simulink model "p2semanti"  (R2020a)
settings: Solver=VariableStepAuto  StartTime=0.0  StopTime=5  RelTol=1e-3
values from neighbouring files (symbols this model uses):
  B = 0.003032    [motorfase_valores.m]
  flux = 0.12    [motorfase_valores.m]
  inddiff = 0.0125    [motorfase_valores.m]
  J = 0.0042    [motorfase_valores.m]
  p = 3    [motorfase_valores.m]
  R = 2.3    [motorfase_valores.m]
undefined symbols (not defined in the file or in its folder): Down, Up
libraries: powerlib x13, eePwmGenerator x1, simulink x1
settings Model: Creator=ryt14  LastModifiedBy=ryt14

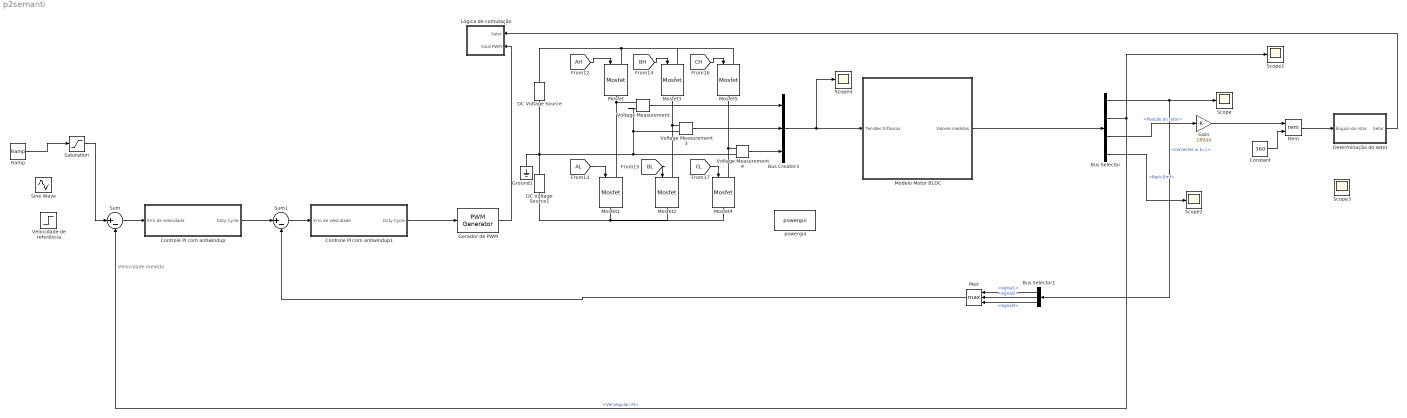
== system p2semanti ==
  note: Velocidade medida
  Bus Creator3 : BusCreator  Inputs=3
  Bus Selector : BusSelector  OutputSignals=Correntes a; b; c,Vel angular: PI,Posição do rotor,Back-Emf
  Bus Selector1 : BusSelector  OutputSignals=signal1,signal2,signal3
  Constant : Constant  Value=360
  Controle PI com antiwindup : Subsystem
  Controle PI com antiwindup1 : Subsystem
  DC Voltage Source : powerlib/Electrical Sources/DC Voltage Source  Amplitude=75  Measurements=None
  DC Voltage Source1 : powerlib/Electrical Sources/DC Voltage Source  Amplitude=75  Measurements=None
  Determinação do setor : Subsystem
  Gain : Gain  Gain=180/pi
  Gerador de PWM : eePwmGenerator/PWM Generator  CarrCount=Up-Down  Tper=0.001  Ts=5e-5
  Ground1 : powerlib/Elements/Ground  LConnTagsString=a
  Lógica de comutação : Subsystem
  Max : MinMax  Function=max  Inputs=3
  Modelo Motor BLDC : Subsystem
  Mosfet{,1..5} (6 alike) : powerlib/Power Electronics/Mosfet  Ron=0.1  Lon=0  Rd=0.01  Vfd=0  IC=0  Rs=1e5  Cs=inf  Measurements=off
  Ramp : simulink/Sources/Ramp  slope=50  start=0  InitialOutput=0
  Rem : Math  Operator=rem  SaturateOnIntegerOverflow=on
  Saturation : Saturate  UpperLimit=100  LowerLimit=0
  Scope{,1..4} (5 alike) : Scope
  Sine Wave : Sin  Amplitude=100  Frequency=pi/5  SampleTime=0
  Sum : Sum  Inputs=|+-
  Sum1 : Sum  Inputs=|+-
  Velocidade de referência : Step  Time=0  After=50  SampleTime=0
  Voltage Measurement : powerlib/Measurements/Voltage Measurement  PhasorSimulation=off  OutputType=Complex  PSBequivalent=0
  Voltage Measurement3 : powerlib/Measurements/Voltage Measurement  PhasorSimulation=off  OutputType=Complex  PSBequivalent=0
  Voltage Measurement4 : powerlib/Measurements/Voltage Measurement  PhasorSimulation=off  OutputType=Complex  PSBequivalent=0
  powergui : powerlib/powergui  Priority=1  SimulationMode=Continuous  SampleTime=50e-6  frequency=60  Iterations=50  frequencyindice=0  Pbase=100e6  ErrMax=1e-4  UnitsV=kV  UnitsW=MW  buscounter=0  FunctionMessages=off  echomessages=off  EnableUseOfTLC=off  CurrentSourceSwitches=off  DisableSnubberDevices=off  DisableRonSwitches=off  DisableVfSwitches=off  DisplayEquations=off  AutomaticDiscreteSolvers=off  SolverType=Tustin/Backward Euler (TBE)  Interpol=off  ExternalGateDelay=off  methode=off  Ts=100  x0status=blocks  SPID=on  SwTol=0  HookPort=off  NonlinearTolerance=1e-4  nMaxIteration=100  ContinueOnMaxIteration=off  RestoreLinks=warning  ResistiveCurrentMeasurement=off  Frange=[0:2:500]  Ylog=off  Xlog=on  ShowGrid=off  save=off  variable=ZData  structure=0  ZoomFFT=off  StartTime=0.0  cycles=1  DisplayStyle=1  fundamental=60  FreqAxis=off  MaxFrequency=1000  frequencyindicesteady=1  RmsSteady=1  display=off
  wires:
  Voltage Measurement3/1 -> Bus Creator3/2
  Voltage Measurement4/1 -> Bus Creator3/3
  Voltage Measurement/1 -> Bus Creator3/1
  Modelo Motor BLDC/1(Valores medidos) -> Bus Selector/1
  Gain/1 -> Rem/1
  Bus Selector/3 -> Gain/1  "<Posição do rotor>"
  Constant/1 -> Rem/2
  Rem/1 -> Determinação do setor/1(Ângulo do rotor)
  Bus Selector/2 -> Sum/2, Scope1/1  "<Vel angular: PI>"
  [AH] -> Mosfet/1
  [BH] -> Mosfet3/1
  [CH] -> Mosfet5/1
  [BL] -> Mosfet2/1
  [CL] -> Mosfet4/1
  [AL] -> Mosfet1/1
  Bus Selector/1 -> Bus Selector1/1, Scope/1  "<Correntes a; b; c>"
  Bus Selector/4 -> Scope2/1  "<Back-Emf>"
  Determinação do setor/1(Setor) -> Lógica de comutação/1(Setor)
  Gerador de PWM/1 -> Lógica de comutação/2(Sinal PWM)
  Sum/1 -> Controle PI com antiwindup/1(Erro de velocidade)
  Bus Creator3/1 -> Scope4/1, Modelo Motor BLDC/1(Tensões trifásicas)
  Bus Selector1/1 -> Max/1  "<signal1>"
  Bus Selector1/2 -> Max/2  "<signal2>"
  Bus Selector1/3 -> Max/3  "<signal3>"
  Sum1/1 -> Controle PI com antiwindup1/1(Erro de velocidade)
  Max/1 -> Sum1/2
  Controle PI com antiwindup/1(Duty Cycle) -> Sum1/1
  Controle PI com antiwindup1/1(Duty Cycle) -> Gerador de PWM/1
  Ramp/1 -> Saturation/1
  Saturation/1 -> Sum/1
  connections:
  Mosfet/RConn1 -- Mosfet1/LConn1 -- Voltage Measurement/LConn1
  Mosfet3/RConn1 -- Mosfet2/LConn1 -- Voltage Measurement3/LConn1
  Mosfet5/RConn1 -- Mosfet4/LConn1 -- Voltage Measurement4/LConn1
  Mosfet/LConn1 -- Mosfet5/LConn1 -- Mosfet3/LConn1 -- DC Voltage Source/RConn1
  DC Voltage Source/LConn1 -- Voltage Measurement4/LConn2 -- Voltage Measurement3/LConn2 -- Voltage Measurement/LConn2 -- Ground1/LConn1 -- DC Voltage Source1/RConn1
  Mosfet4/RConn1 -- Mosfet2/RConn1 -- DC Voltage Source1/LConn1 -- Mosfet1/RConn1

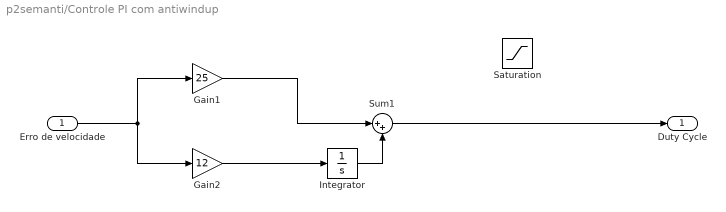
== system p2semanti/Controle PI com antiwindup ==
  Erro de velocidade : Inport
  Gain1 : Gain  Gain=25
  Gain2 : Gain  Gain=12
  Integrator : Integrator
  Saturation : Saturate
  Sum1 : Sum  Inputs=|++
  Duty Cycle : Outport
  wires:
  Integrator/1 -> Sum1/2
  Gain1/1 -> Sum1/1
  Erro de velocidade/1 -> Gain1/1, Gain2/1
  Sum1/1 -> Duty Cycle/1
  Gain2/1 -> Integrator/1

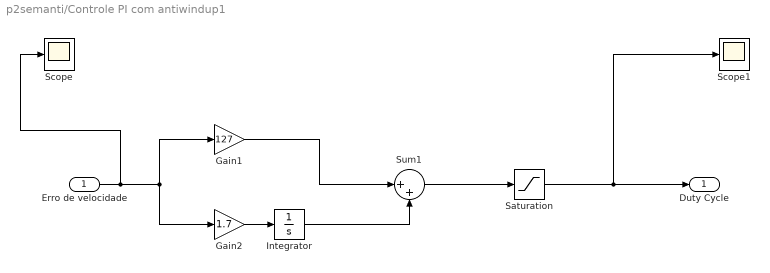
== system p2semanti/Controle PI com antiwindup1 ==
  Erro de velocidade : Inport
  Gain1 : Gain  Gain=127
  Gain2 : Gain  Gain=1.7
  Integrator : Integrator
  Saturation : Saturate  UpperLimit=1  LowerLimit=0
  Scope : Scope
  Scope1 : Scope
  Sum1 : Sum  Inputs=|++
  Duty Cycle : Outport
  wires:
  Sum1/1 -> Saturation/1
  Erro de velocidade/1 -> Scope/1, Gain1/1, Gain2/1
  Saturation/1 -> Scope1/1, Duty Cycle/1
  Gain2/1 -> Integrator/1
  Integrator/1 -> Sum1/2
  Gain1/1 -> Sum1/1

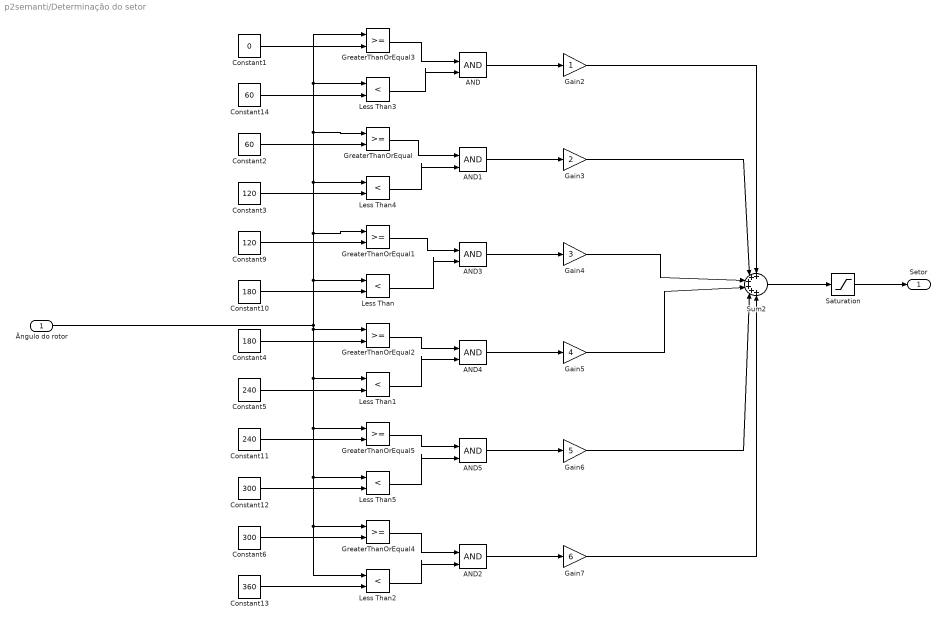
== system p2semanti/Determinação do setor ==
  Ângulo do rotor : Inport
  AND{,1..5} (6 alike) : Logic  IconShape=distinctive  AllPortsSameDT=off  OutDataTypeStr=boolean
  Constant1 : Constant  Value=0
  Constant10 : Constant  Value=180
  Constant11 : Constant  Value=240
  Constant12 : Constant  Value=300
  Constant13 : Constant  Value=360
  Constant14 : Constant  Value=60
  Constant2 : Constant  Value=60
  Constant3 : Constant  Value=120
  Constant4 : Constant  Value=180
  Constant5 : Constant  Value=240
  Constant6 : Constant  Value=300
  Constant9 : Constant  Value=120
  Gain2 : Gain
  Gain3 : Gain  Gain=2
  Gain4 : Gain  Gain=3
  Gain5 : Gain  Gain=4
  Gain6 : Gain  Gain=5
  Gain7 : Gain  Gain=6
  GreaterThanOrEqual{,1..5} (6 alike) : RelationalOperator  OutDataTypeStr=boolean  RndMeth=Simplest
  Less Than{,1..5} (6 alike) : RelationalOperator  Operator=<  OutDataTypeStr=boolean  RndMeth=Simplest
  Saturation : Saturate  UpperLimit=6  LowerLimit=1
  Sum2 : Sum  Inputs=++++++
  Setor : Outport
  wires:
  Ângulo do rotor/1 -> Less Than/1, GreaterThanOrEqual1/1, GreaterThanOrEqual/1, GreaterThanOrEqual3/1, Less Than3/1, Less Than4/1, Less Than2/1, GreaterThanOrEqual4/1, Less Than5/1, GreaterThanOrEqual5/1, Less Than1/1, GreaterThanOrEqual2/1
  Less Than1/1 -> AND4/2
  Gain2/1 -> Sum2/1
  Sum2/1 -> Saturation/1
  Constant1/1 -> GreaterThanOrEqual3/2
  Constant9/1 -> GreaterThanOrEqual1/2
  Gain4/1 -> Sum2/3
  Gain5/1 -> Sum2/4
  AND/1 -> Gain2/1
  Constant13/1 -> Less Than2/2
  Constant2/1 -> GreaterThanOrEqual/2
  AND4/1 -> Gain5/1
  AND1/1 -> Gain3/1
  Less Than5/1 -> AND5/2
  Less Than/1 -> AND3/2
  GreaterThanOrEqual1/1 -> AND3/1
  Constant4/1 -> GreaterThanOrEqual2/2
  Gain3/1 -> Sum2/2
  Less Than2/1 -> AND2/2
  GreaterThanOrEqual5/1 -> AND5/1
  GreaterThanOrEqual/1 -> AND1/1
  Gain6/1 -> Sum2/5
  AND2/1 -> Gain7/1
  AND5/1 -> Gain6/1
  Less Than3/1 -> AND/2
  Constant11/1 -> GreaterThanOrEqual5/2
  Constant12/1 -> Less Than5/2
  Constant3/1 -> Less Than4/2
  Constant5/1 -> Less Than1/2
  Saturation/1 -> Setor/1
  AND3/1 -> Gain4/1
  Constant14/1 -> Less Than3/2
  GreaterThanOrEqual2/1 -> AND4/1
  Less Than4/1 -> AND1/2
  Constant6/1 -> GreaterThanOrEqual4/2
  Constant10/1 -> Less Than/2
  GreaterThanOrEqual4/1 -> AND2/1
  Gain7/1 -> Sum2/6
  GreaterThanOrEqual3/1 -> AND/1

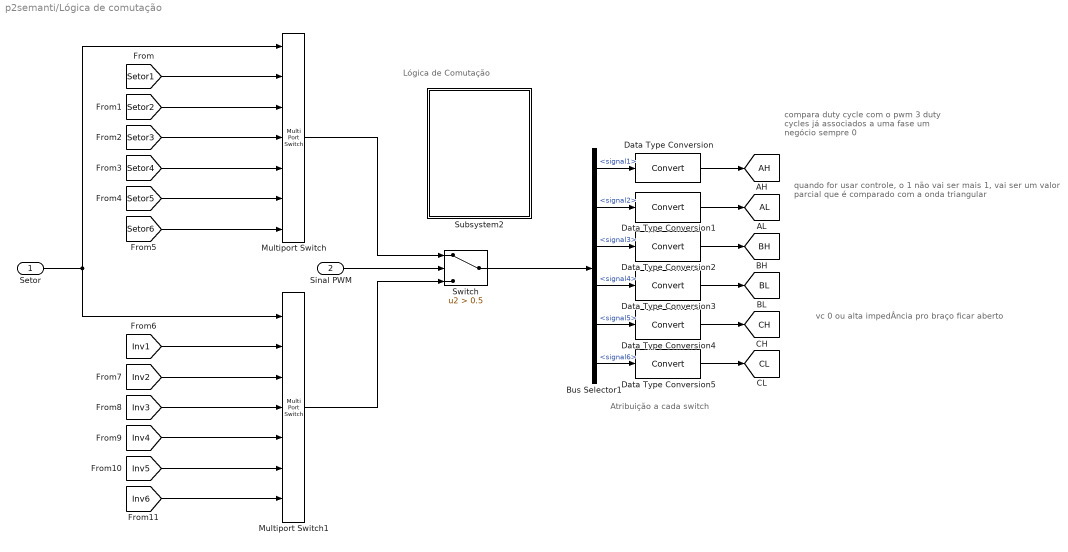
== system p2semanti/Lógica de comutação ==
  note: vc 0 ou alta impedÂncia pro braço ficar aberto
  note: quando for usar controle, o 1 não vai ser mais 1,
      | vai ser um valor parcial que é comparado com a onda triangular
  note: compara duty cycle com o pwm
      | 3 duty cycles já associados a uma fase
      | um negócio sempre 0
  note: Atribuição a cada switch
  note: Lógica de Comutação
  Setor : Inport
  Sinal PWM : Inport  Port=2
  Bus Selector1 : BusSelector  OutputSignals=signal1,signal2,signal3,signal4,signal5,signal6
  Data Type Conversion{,1..5} (6 alike) : DataTypeConversion
  Multiport Switch : MultiPortSwitch  Inputs=6
  Multiport Switch1 : MultiPortSwitch  Inputs=6
  Subsystem2 : Subsystem
  Switch : Switch  Criteria=u2 > Threshold  Threshold=0.5
  tag scope: AH=global, AL=global, BH=global, BL=global, CH=global, CL=global
  wires:
  [Inv4] -> Multiport Switch1/5
  Data Type Conversion5/1 -> [CL]
  [Setor1] -> Multiport Switch/2
  Bus Selector1/2 -> Data Type Conversion1/1  "<signal2>"
  Bus Selector1/4 -> Data Type Conversion3/1  "<signal4>"
  Data Type Conversion4/1 -> [CH]
  [Setor2] -> Multiport Switch/3
  [Inv1] -> Multiport Switch1/2
  Data Type Conversion1/1 -> [AL]
  Bus Selector1/3 -> Data Type Conversion2/1  "<signal3>"
  [Setor3] -> Multiport Switch/4
  [Inv3] -> Multiport Switch1/4
  Data Type Conversion3/1 -> [BL]
  [Setor5] -> Multiport Switch/6
  Switch/1 -> Bus Selector1/1
  Multiport Switch/1 -> Switch/1
  Bus Selector1/1 -> Data Type Conversion/1  "<signal1>"
  [Inv5] -> Multiport Switch1/6
  [Inv6] -> Multiport Switch1/7
  Bus Selector1/6 -> Data Type Conversion5/1  "<signal6>"
  [Inv2] -> Multiport Switch1/3
  Setor/1 -> Multiport Switch/1, Multiport Switch1/1
  Data Type Conversion/1 -> [AH]
  Bus Selector1/5 -> Data Type Conversion4/1  "<signal5>"
  [Setor4] -> Multiport Switch/5
  Data Type Conversion2/1 -> [BH]
  Multiport Switch1/1 -> Switch/3
  [Setor6] -> Multiport Switch/7
  Sinal PWM/1 -> Switch/2

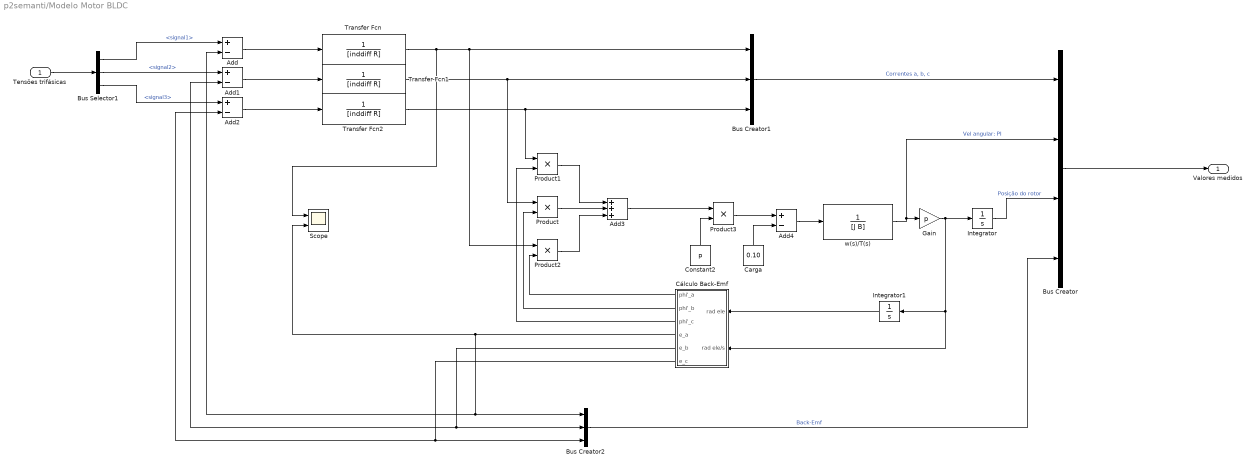
== system p2semanti/Modelo Motor BLDC ==
  Tensões trifásicas : Inport
  Add{,1..2,4} (4 alike) : Sum  Inputs=+-
  Add3 : Sum  Inputs=+++
  Bus Creator : BusCreator  Inputs=4
  Bus Creator1 : BusCreator  Inputs=3
  Bus Creator2 : BusCreator  Inputs=3
  Bus Selector1 : BusSelector  OutputSignals=signal1,signal2,signal3
  Carga : Constant  Value=0.10
  Constant2 : Constant  Value=p
  Cálculo Back-Emf : Subsystem
  Gain : Gain  Gain=p
  Integrator : Integrator
  Integrator1 : Integrator
  Product : Product
  Product1 : Product
  Product2 : Product
  Product3 : Product  Inputs=**
  Scope : Scope  NumInputPorts=2
  Transfer Fcn : TransferFcn  Denominator=[inddiff R]
  Transfer Fcn1 : TransferFcn  Denominator=[inddiff R]
  Transfer Fcn2 : TransferFcn  Denominator=[inddiff R]
  w(s)/T(s) : TransferFcn  Denominator=[J B]
  Valores medidos : Outport
  wires:
  Add/1 -> Transfer Fcn/1
  Add2/1 -> Transfer Fcn2/1
  Carga/1 -> Add4/2
  Bus Selector1/2 -> Add1/1  "<signal2>"
  Bus Creator1/1 -> Bus Creator/1  "Correntes a, b, c"
  Add1/1 -> Transfer Fcn1/1
  Transfer Fcn1/1 -> Bus Creator1/2, Product/1
  Product3/1 -> Add4/1
  Bus Selector1/1 -> Add/1  "<signal1>"
  Transfer Fcn2/1 -> Bus Creator1/3, Product1/1
  Add4/1 -> w(s)/T(s)/1
  Transfer Fcn/1 -> Scope/1, Bus Creator1/1, Product2/1
  Bus Selector1/3 -> Add2/1  "<signal3>"
  Bus Creator2/1 -> Bus Creator/4  "Back-Emf"
  Product/1 -> Add3/2
  Tensões trifásicas/1 -> Bus Selector1/1
  Gain/1 -> Integrator/1, Cálculo Back-Emf/2(rad ele/s), Integrator1/1
  Integrator/1 -> Bus Creator/3  "Posição do rotor"
  Bus Creator/1 -> Valores medidos/1
  Add3/1 -> Product3/1
  Constant2/1 -> Product3/2
  w(s)/T(s)/1 -> Gain/1, Bus Creator/2  "Vel angular: PI"
  Cálculo Back-Emf/5(e_b) -> Add1/2, Bus Creator2/2
  Cálculo Back-Emf/6(e_c) -> Add2/2, Bus Creator2/3
  Cálculo Back-Emf/4(e_a) -> Scope/2, Add/2, Bus Creator2/1
  Integrator1/1 -> Cálculo Back-Emf/1(rad ele)
  Cálculo Back-Emf/1(phi'_a) -> Product2/2
  Cálculo Back-Emf/2(phi'_b) -> Product/2
  Cálculo Back-Emf/3(phi'_c) -> Product1/2
  Product2/1 -> Add3/3
  Product1/1 -> Add3/1

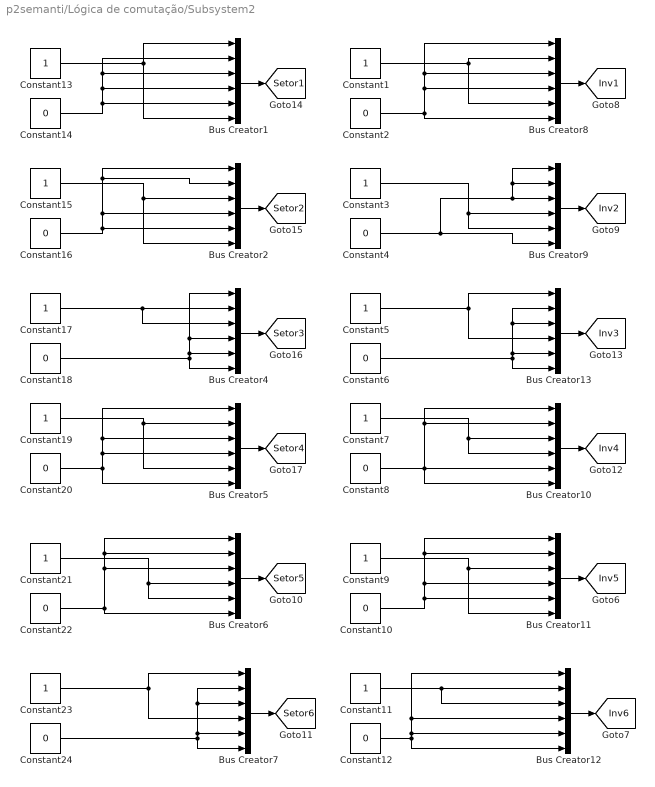
== system p2semanti/Lógica de comutação/Subsystem2 ==
  Bus Creator{1..2,4..13} (12 alike) : BusCreator  Inputs=6
  Constant{1,3,5,7,9,11,13,15,17,19,21,23} (12 alike) : Constant
  Constant{2,4,6,8,10,12,14,16,18,20,22,24} (12 alike) : Constant  Value=0
  tag scope: Inv1=global, Inv2=global, Inv3=global, Inv4=global, Inv5=global, Inv6=global, Setor1=global, Setor2=global, Setor3=global, Setor4=global, Setor5=global, Setor6=global
  wires:
  Constant13/1 -> Bus Creator1/6, Bus Creator1/1
  Bus Creator12/1 -> [Inv6]
  Constant24/1 -> Bus Creator7/6, Bus Creator7/5, Bus Creator7/3, Bus Creator7/2
  Bus Creator9/1 -> [Inv2]
  Constant16/1 -> Bus Creator2/4, Bus Creator2/2, Bus Creator2/1, Bus Creator2/5
  Constant6/1 -> Bus Creator13/6, Bus Creator13/3, Bus Creator13/2, Bus Creator13/5
  Constant1/1 -> Bus Creator8/2, Bus Creator8/5
  Constant4/1 -> Bus Creator9/1, Bus Creator9/2, Bus Creator9/3, Bus Creator9/6
  Bus Creator7/1 -> [Setor6]
  Constant18/1 -> Bus Creator4/6, Bus Creator4/5, Bus Creator4/4, Bus Creator4/1
  Constant12/1 -> Bus Creator12/5, Bus Creator12/1, Bus Creator12/4, Bus Creator12/6
  Constant23/1 -> Bus Creator7/4, Bus Creator7/1
  Constant7/1 -> Bus Creator10/4, Bus Creator10/3
  Constant10/1 -> Bus Creator11/1, Bus Creator11/2, Bus Creator11/4, Bus Creator11/5
  Constant14/1 -> Bus Creator1/4, Bus Creator1/3, Bus Creator1/2, Bus Creator1/5
  Constant3/1 -> Bus Creator9/5, Bus Creator9/4
  Constant15/1 -> Bus Creator2/6, Bus Creator2/3
  Bus Creator5/1 -> [Setor4]
  Constant8/1 -> Bus Creator10/2, Bus Creator10/1, Bus Creator10/5, Bus Creator10/6
  Constant2/1 -> Bus Creator8/6, Bus Creator8/3, Bus Creator8/1, Bus Creator8/4
  Bus Creator6/1 -> [Setor5]
  Constant17/1 -> Bus Creator4/3, Bus Creator4/2
  Bus Creator4/1 -> [Setor3]
  Constant19/1 -> Bus Creator5/2, Bus Creator5/5
  Constant5/1 -> Bus Creator13/4, Bus Creator13/1
  Bus Creator11/1 -> [Inv5]
  Bus Creator1/1 -> [Setor1]
  Bus Creator8/1 -> [Inv1]
  Bus Creator2/1 -> [Setor2]
  Bus Creator10/1 -> [Inv4]
  Constant21/1 -> Bus Creator6/5, Bus Creator6/4
  Bus Creator13/1 -> [Inv3]
  Constant22/1 -> Bus Creator6/6, Bus Creator6/3, Bus Creator6/2, Bus Creator6/1
  Constant20/1 -> Bus Creator5/6, Bus Creator5/4, Bus Creator5/1, Bus Creator5/3
  Constant9/1 -> Bus Creator11/6, Bus Creator11/3
  Constant11/1 -> Bus Creator12/3, Bus Creator12/2

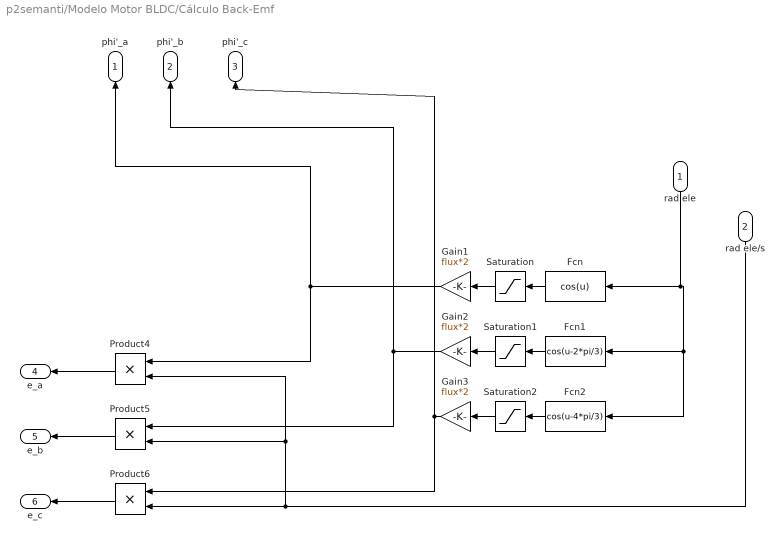
== system p2semanti/Modelo Motor BLDC/Cálculo Back-Emf ==
  rad ele : Inport
  rad ele/s : Inport  Port=2
  Fcn : Fcn  Expr=cos(u)
  Fcn1 : Fcn  Expr=cos(u-2*pi/3)
  Fcn2 : Fcn  Expr=cos(u-4*pi/3)
  Gain1 : Gain  Gain=flux*2
  Gain2 : Gain  Gain=flux*2
  Gain3 : Gain  Gain=flux*2
  Product4 : Product
  Product5 : Product
  Product6 : Product
  Saturation : Saturate
  Saturation1 : Saturate
  Saturation2 : Saturate
  phi'_a : Outport
  phi'_b : Outport  Port=2
  phi'_c : Outport  Port=3
  e_a : Outport  Port=4
  e_b : Outport  Port=5
  e_c : Outport  Port=6
  wires:
  Saturation2/1 -> Gain3/1
  Fcn/1 -> Saturation/1
  Fcn2/1 -> Saturation2/1
  Gain3/1 -> phi'_c/1, Product6/1
  Gain2/1 -> phi'_b/1, Product5/1
  Saturation/1 -> Gain1/1
  Gain1/1 -> phi'_a/1, Product4/1
  Fcn1/1 -> Saturation1/1
  Saturation1/1 -> Gain2/1
  rad ele/1 -> Fcn2/1, Fcn1/1, Fcn/1
  rad ele/s/1 -> Product4/2, Product5/2, Product6/2
  Product6/1 -> e_c/1
  Product4/1 -> e_a/1
  Product5/1 -> e_b/1
